simulink model "abs_dbw"  (R2020b)
settings: Solver=VariableStepAuto  StartTime=0.0  StopTime=50000  FixedStep=0.01  RelTol=1
undefined symbols (not defined in the file): g, Jw, m, mu, Rw, slip, Vi
libraries: pid_lib x1
settings Model: DataDictionary=abs_dd.sldd  Creator=ADITYA NIMBALKAR  LastModifiedBy=K E S SRINIVAS
settings DataIOCC: SaveFormat=StructureWithTime
settings OptimizationCC: BlockReduction=off  DefaultParameterBehavior=Inlined  InlineInvariantSignals=on  EnhancedBackFolding=on  PassReuseOutputArgsThreshold=0  EfficientFloat2IntCast=on  OptimizeBlockOrder=speed  DifferentSizesBufferReuse=on  OptimizationCustomize=off
settings DebuggingCC: SignalInfNanChecking=error  ReadBeforeWriteMsg=EnableAllAsError  WriteAfterWriteMsg=EnableAllAsError  WriteAfterReadMsg=EnableAllAsError  AlgebraicLoopMsg=error  ArtificialAlgebraicLoopMsg=error  SaveWithDisabledLinksMsg=error  SaveWithParameterizedLinksMsg=error  BlockPriorityViolationMsg=error  InheritedTsInSrcMsg=error  SingleTaskRateTransMsg=error  TasksWithSamePriorityMsg=error  SigSpecEnsureSampleTimeMsg=error  CheckMatrixSingularityMsg=error  IntegerOverflowMsg=error  ParameterUnderflowMsg=error  ParameterPrecisionLossMsg=error  ParameterTunabilityLossMsg=error  UnderSpecifiedDataTypeMsg=error  UnnecessaryDatatypeConvMsg=warning  VectorMatrixConversionMsg=error  SignalLabelMismatchMsg=error  UnconnectedInputMsg=error  UnconnectedOutputMsg=error  UnconnectedLineMsg=error  SFcnCompatibilityMsg=error  FrameProcessingCompatibilityMsg=warning  UniqueDataStoreMsg=error  BusObjectLabelMismatch=error  RootOutportRequireBusObject=error  AssertControl=DisableAll  ModelReferenceIOMsg=error  ModelReferenceIOMismatchMessage=error  UnknownTsInhSupMsg=error  ModelReferenceDataLoggingMessage=error  StateNameClashWarn=warning  NonCurrentReleaseOperatingPointMsg=warning  StrictBusMsg=ErrorOnBusTreatedAsVector  NonBusSignalsTreatedAsBus=error  SFInvalidInputDataAccessInChartInitDiag=error  SFTransitionOutsideNaturalParentDiag=error  SFUnreachableExecutionPathDiag=error  SFUndirectedBroadcastEventsDiag=error  SFTransitionActionBeforeConditionDiag=error  IntegerSaturationMsg=error
settings HardwareCC: TargetBitPerPointer=64  TargetBitPerSizeT=64  TargetBitPerPtrDiffT=64  TargetLongLongMode=on  TargetIntDivRoundTo=Zero  TargetEndianess=LittleEndian  TargetWordSize=64  TargetHWDeviceType=MATLAB Host  ProdEqTarget=off
settings ModelReferenceCC: ModelReferenceNumInstancesAllowed=Single
settings SFSimCC: MATLABDynamicMemAlloc=off
settings RTWCC: Description=Rapid Simulation Target  SystemTargetFile=rsim.tlc  TemplateMakefile=rsim_default_tmf  GenerateReport=on  LaunchReport=on
settings CodeAppCC: ForceParamTrailComments=on  OperatorAnnotations=on  MangleLength=4
settings RSimTargetCC: TargetLangStandard=C99 (ISO)

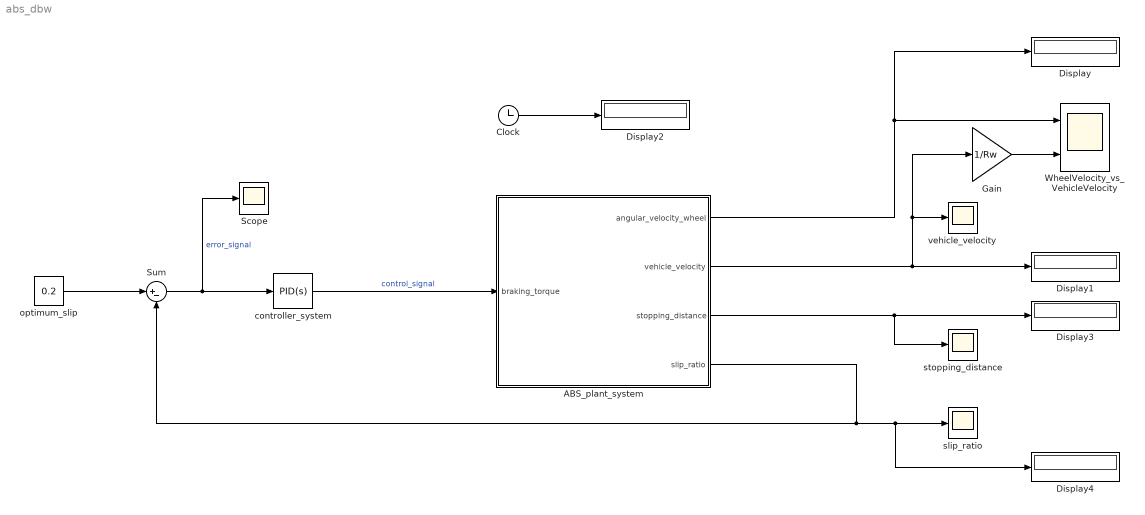
== system abs_dbw ==
  ABS_plant_system : Subsystem
  Clock : Clock
  Display{,1..4} (5 alike) : Display
  Gain : Gain  Gain=1/Rw
  Scope : Scope
  Sum : Sum  Inputs=|+-
  WheelVelocity_vs_VehicleVelocity : Scope  NumInputPorts=2
  controller_system : pid_lib/PID Controller  Controller=PID  Form=Parallel  TimeDomain=Continuous-time  UseExternalTs=off  SampleTime=-1  IntegratorMethod=Forward Euler  FilterMethod=Forward Euler  ControllerParametersSource=internal  P=250  I=10  D=5  UseFilter=on  N=100  TunerSelectOption=Transfer Function Based (PID Tuner App)  InitialConditionSource=internal  InitialConditionForIntegrator=0  InitialConditionForFilter=0  DifferentiatorICPrevScaledInput=0  ExternalReset=none  TrackingMode=off  Kt=1  LimitOutput=off  SatLimitsSource=internal  UpperSaturationLimit=inf  LowerSaturationLimit=-inf  LinearizeAsGain=on  AntiWindupMode=none  Kb=1  POutMin=[]  POutMax=[]  IOutMin=[]  IOutMax=[]  DOutMin=[]  DOutMax=[]  NOutMin=[]  NOutMax=[]  SumOutMin=[]  SumOutMax=[]  SaturationOutMin=[]  SaturationOutMax=[]  PParamMin=[]  PParamMax=[]  IParamMin=[]  IParamMax=[]  DParamMin=[]  DParamMax=[]  NParamMin=[]  NParamMax=[]  KbParamMin=[]  KbParamMax=[]  KtParamMin=[]  KtParamMax=[]  KbOutMin=[]  KbOutMax=[]  KtOutMin=[]  KtOutMax=[]  IntegratorOutMin=[]  IntegratorOutMax=[]  FilterOutMin=[]  FilterOutMax=[]  SumI1OutMin=[]  SumI1OutMax=[]  SumI2OutMin=[]  SumI2OutMax=[]  SumI3OutMin=[]  SumI3OutMax=[]  SumI4OutMin=[]  SumI4OutMax=[]  SumDOutMin=[]  SumDOutMax=[]  DifferentiatorOutMin=[]  DifferentiatorOutMax=[]  FilterDiffOutCoefMin=[]  FilterDiffOutCoefMax=[]  ReciprocalOutMin=[]  ReciprocalOutMax=[]  SumDenOutMin=[]  SumDenOutMax=[]  SumNumOutMin=[]  SumNumOutMax=[]  DivideOutMin=[]  DivideOutMax=[]  UdiffTsProdOutMin=[]  UdiffTsProdOutMax=[]  NTsProdOutMin=[]  NTsProdOutMax=[]  UintegralTsProdOutMin=[]  UintegralTsProdOutMax=[]  UngainTsProdOutMin=[]  UngainTsProdOutMax=[]  IntegratorContinuousStateAttributes=''  IntegratorStateMustResolveToSignalObject=off  IntegratorRTWStateStorageClass=Auto  FilterContinuousStateAttributes=''  FilterStateMustResolveToSignalObject=off  FilterRTWStateStorageClass=Auto  ParallelPVariant=InternalParameters  IdealPVariant=Disabled  IVariant=InternalParameters  DVariant=InternalParameters  IntegratorVariant=Continuous  SatVariant=Disabled  AWVariant=Passthrough  PCopyVariant=Disabled  TRVariant=Disabled  FdbkBlocksVariant=Forward  IdealPFdbkVariant=Disabled  SatFdbkVariant=Disabled  DerivativeFilterVariant=ContFilter  NVariant=InternalParameters  NCopyVariant=Disabled  FilterICVariant=InternalICsFilter  IntegratorICVariant=InternalICs  ExternalResetVariant=Disabled  TRSumVariant=Passthrough  SumFdbkVariant=Disabled  SumVariant=Sum_PID  TsampFilterVariant=InternalTs  TsampNgainVariant=Passthrough  TsampIntegralVariant=Passthrough  ExternalSaturationOutDataTypeStr=Inherit: Same as second input
  optimum_slip : Constant  Value=0.2  OutDataTypeStr=double
  slip_ratio : Scope
  stopping_distance : Scope
  vehicle_velocity : Scope
  wires:
  optimum_slip/1 -> Sum/1
  Sum/1 -> Scope/1, controller_system/1  "error_signal"
  ABS_plant_system/4(slip_ratio) -> Sum/2, Display4/1, slip_ratio/1
  Clock/1 -> Display2/1
  controller_system/1 -> ABS_plant_system/1(braking_torque)  "control_signal"
  ABS_plant_system/3(stopping_distance) -> stopping_distance/1, Display3/1
  ABS_plant_system/2(vehicle_velocity) -> Gain/1, vehicle_velocity/1, Display1/1
  ABS_plant_system/1(angular_velocity_wheel) -> Display/1, WheelVelocity_vs_VehicleVelocity/1
  Gain/1 -> WheelVelocity_vs_VehicleVelocity/2

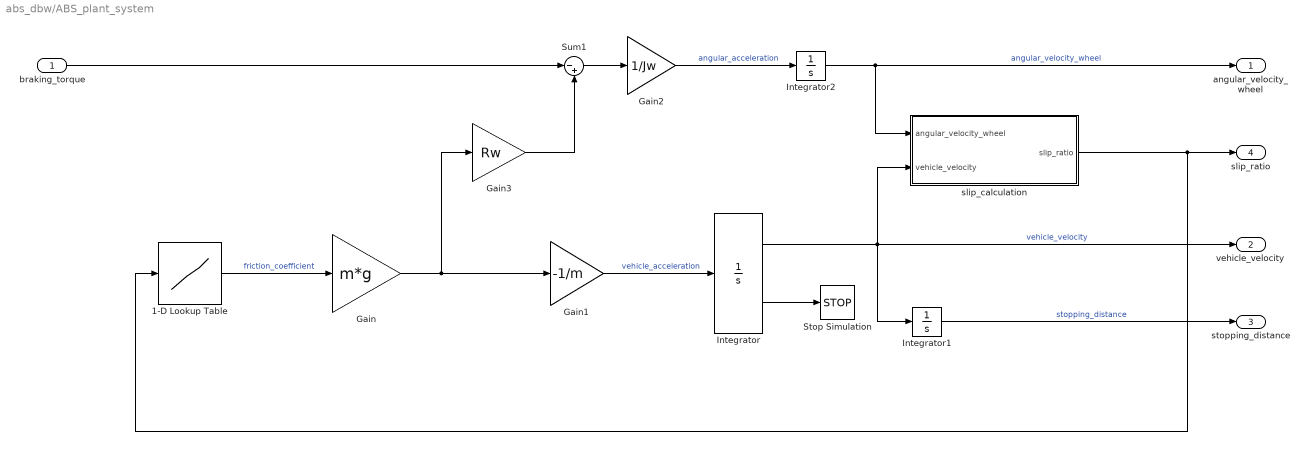
== system abs_dbw/ABS_plant_system ==
  braking_torque : Inport
  1-D Lookup Table : Lookup_n-D  NumberOfTableDimensions=1  BreakpointsForDimension1=slip  Table=mu  InternalRulePriority=Speed  RndMeth=Simplest  SaturateOnIntegerOverflow=on
  Gain : Gain  Gain=m*g
  Gain1 : Gain  Gain=-1/m
  Gain2 : Gain  Gain=1/Jw
  Gain3 : Gain  Gain=Rw
  Integrator : Integrator  InitialCondition=Vi  LimitOutput=on  UpperSaturationLimit=1000  LowerSaturationLimit=0  ShowSaturationPort=on
  Integrator1 : Integrator
  Integrator2 : Integrator  InitialCondition=Vi/Rw  LimitOutput=on  UpperSaturationLimit=1000  LowerSaturationLimit=0
  Stop Simulation : Stop
  Sum1 : Sum  Inputs=|-+
  slip_calculation : Subsystem
  angular_velocity_wheel : Outport
  vehicle_velocity : Outport  Port=2
  stopping_distance : Outport  Port=3
  slip_ratio : Outport  Port=4
  wires:
  Gain1/1 -> Integrator/1  "vehicle_acceleration"
  Integrator/1 -> Integrator1/1, vehicle_velocity/1, slip_calculation/2(vehicle_velocity)  "vehicle_velocity"
  Integrator/2 -> Stop Simulation/1
  Integrator1/1 -> stopping_distance/1  "stopping_distance"
  Gain2/1 -> Integrator2/1  "angular_acceleration"
  Sum1/1 -> Gain2/1
  Gain3/1 -> Sum1/2
  1-D Lookup Table/1 -> Gain/1  "friction_coefficient"
  braking_torque/1 -> Sum1/1
  Integrator2/1 -> angular_velocity_wheel/1, slip_calculation/1(angular_velocity_wheel)  "angular_velocity_wheel"
  Gain/1 -> Gain1/1, Gain3/1
  slip_calculation/1(slip_ratio) -> 1-D Lookup Table/1, slip_ratio/1

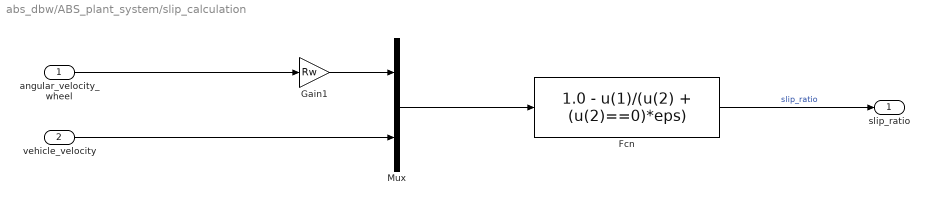
== system abs_dbw/ABS_plant_system/slip_calculation ==
  angular_velocity_wheel : Inport
  vehicle_velocity : Inport  Port=2
  Fcn : Fcn  Expr=1.0 - u(1)/(u(2) + (u(2)==0)*eps)
  Gain1 : Gain  Gain=Rw
  Mux : Mux  Inputs=2
  slip_ratio : Outport
  wires:
  vehicle_velocity/1 -> Mux/2
  angular_velocity_wheel/1 -> Gain1/1
  Fcn/1 -> slip_ratio/1  "slip_ratio"
  Mux/1 -> Fcn/1
  Gain1/1 -> Mux/1
